simulink model "MVDR_example_hdl_4x4_systolic"  (R2020a)
settings: Solver=FixedStepDiscrete  StartTime=0.0  StopTime=stoptime  RelTol=1e-3
InitFcn:
  | model_init
values from neighbouring files (symbols this model uses):
  BackSubstitutePrototype = fi(0, matrixdivbacksub_dt)    [model_init.m]
  matrixDivDelay = NumberOfCORDICIterations*10 + 86    [model_init.m]
  movavg_bitshift = nextpow2(sqrt(windowSize))    [model_init.m]
  mvdrPipelineDelay = covMatDelay+movAvgDelay+matrixDivDelay+normResponseDelay    [model_init.m]
  numArrayElements = 4    [model_init.m]
  NumberOfCORDICIterations = matrixdivin_dt.WordLength - 1    [model_init.m]
  srcAngles = [20 60]    [model_init.m]
  sv = step(steeringVector,fc,[scanAngle; 0])    [model_init.m]
  Ts = 1/fs    (= 7.8125e-09)    [model_init.m]
  windowSize = 1024    [model_init.m]
libraries: hdlsllib x249, simulink x44, commfilt2 x4, commrfcorlib x3, commsync2 x3, commrflib2 x2, commrandsrc3 x2, phasedtxrxlib x2, commdigbbndcpm2 x1, dspsolvers x1, embreciprocals x1, commdigbbndpm3 x1
(part 1 of 11)
Description:
  | MVDR HDL 4x4 systolic testbench
settings Model: DataTypeOverride=Off  Creator=The MathWorks, Inc.  LastModifiedBy=tmealey
settings DataIOCC: LimitDataPoints=on  SaveFormat=Array  SaveOutput=off  SaveTime=off  ReturnWorkspaceOutputs=off
settings OptimizationCC: BlockReduction=off  ConditionallyExecuteInputs=off  DefaultParameterBehavior=Inlined  LifeSpan=inf
settings DebuggingCC: ReadBeforeWriteMsg=DisableAll  WriteAfterWriteMsg=DisableAll  WriteAfterReadMsg=DisableAll  AlgebraicLoopMsg=error  UnderspecifiedInitializationDetection=Classic  MergeDetectMultiDrivingBlocksExec=none  SolverPrmCheckMsg=warning  SingleTaskRateTransMsg=error  ParameterPrecisionLossMsg=none  AllowSymbolicDim=off  SFUnexpectedBacktrackingDiag=warning  SFNoUnconditionalDefaultTransitionDiag=warning  SFExecutionAtInitializationDiag=none  ArithmeticOperatorsInVariantConditions=warning
settings HardwareCC: ProdBitPerPointer=32  ProdBitPerSizeT=32  ProdBitPerPtrDiffT=32  ProdLargestAtomicFloat=None  ProdIntDivRoundTo=Undefined  ProdEndianess=Unspecified  ProdWordSize=32  ProdHWDeviceType=ASIC/FPGA->ASIC/FPGA  TargetBitPerPointer=64  TargetBitPerSizeT=64  TargetBitPerPtrDiffT=64  TargetLongLongMode=on  TargetIntDivRoundTo=Zero  TargetEndianess=LittleEndian  TargetWordSize=64  TargetHWDeviceType=Custom Processor->MATLAB Host Computer  ProdEqTarget=off
settings ModelReferenceCC: PropagateSignalLabelsOutOfModel=off
settings SFSimCC: SimUseLocalCustomCode=off  CustomCodeUndefinedFunction=UseInterfaceOnly
settings RTWCC: RTWUseLocalCustomCode=off
settings CodeAppCC: StateflowObjectComments=on
settings GRTTargetCC: TargetLangStandard=C89/C90 (ANSI)
settings ConfigComp: CovMetricSettings=dw  CovHtmlReporting=on  CovSaveCumulativeToWorkspaceVar=on  CovSaveSingleToWorkspaceVar=on  CovExternalEMLEnable=off  CovSFcnEnable=off

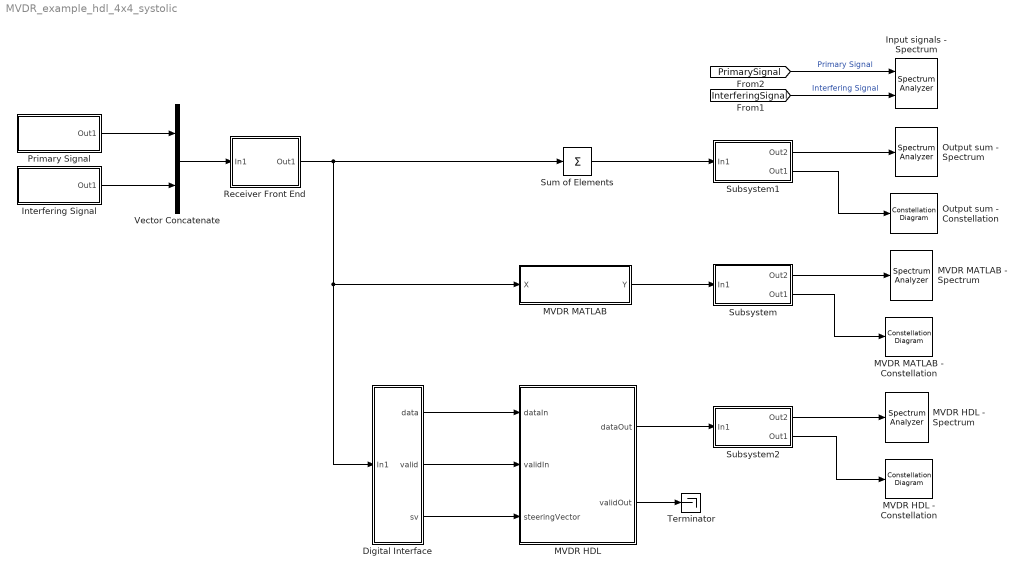
== system MVDR_example_hdl_4x4_systolic ==
  Digital Interface : Subsystem
  Input signals - Spectrum : SpectrumAnalyzer  NumInputPorts=2
  Interfering Signal : Subsystem
      mask Display: disp('Interfering\nSignal')
  MVDR HDL : Subsystem
  MVDR HDL - Constellation : ConstellationDiagram
  MVDR HDL - Spectrum : SpectrumAnalyzer
  MVDR MATLAB : Subsystem
  MVDR MATLAB - Constellation : ConstellationDiagram
  MVDR MATLAB - Spectrum : SpectrumAnalyzer
  Output sum - Constellation : ConstellationDiagram
  Output sum - Spectrum : SpectrumAnalyzer
  Primary Signal : Subsystem
      mask Display: disp('Primary\nSignal')
  Receiver Front End : Subsystem
  Subsystem : Subsystem
  Subsystem1 : Subsystem
  Subsystem2 : Subsystem
  Sum of Elements : Sum  Inputs=+  CollapseMode=Specified dimension  CollapseDim=2
  Terminator : Terminator
  Vector Concatenate : Concatenate  Mode=Multidimensional array  ConcatenateDimension=2
  wires:
  MVDR HDL/2(validOut) -> Terminator/1
  MVDR MATLAB/1(Y) -> Subsystem/1(In1)
  Interfering Signal/1(Out1) -> Vector Concatenate/2
  Primary Signal/1(Out1) -> Vector Concatenate/1
  [InterferingSignal] -> Input signals - Spectrum/2  "Interfering Signal"
  Subsystem/2(Out1) -> MVDR MATLAB - Constellation/1
  Subsystem/1(Out2) -> MVDR MATLAB - Spectrum/1
  Sum of Elements/1 -> Subsystem1/1(In1)
  Subsystem1/1(Out2) -> Output sum - Spectrum/1
  Subsystem1/2(Out1) -> Output sum - Constellation/1
  MVDR HDL/1(dataOut) -> Subsystem2/1(In1)
  Subsystem2/1(Out2) -> MVDR HDL - Spectrum/1
  Subsystem2/2(Out1) -> MVDR HDL - Constellation/1
  [PrimarySignal] -> Input signals - Spectrum/1  "Primary Signal"
  Digital Interface/1(data) -> MVDR HDL/1(dataIn)
  Digital Interface/2(valid) -> MVDR HDL/2(validIn)
  Digital Interface/3(sv) -> MVDR HDL/3(steeringVector)
  Receiver Front End/1(Out1) -> MVDR MATLAB/1(X), Digital Interface/1(In1), Sum of Elements/1
  Vector Concatenate/1 -> Receiver Front End/1(In1)

== system MVDR_example_hdl_4x4_systolic/Digital Interface ==
  In1 : Inport
  Constant1 : Constant  Value=true  SampleTime=-1
  Constant2 : Constant  Value=sv  SampleTime=-1
  Data Type Conversion : DataTypeConversion  OutDataTypeStr=sv_dt
  Input DTC : Subsystem
  Reshape : Reshape  OutputDimensionality=Column vector (2-D)
  Unbuffer : Unbuffer
  data : Outport
  valid : Outport  Port=2
  sv : Outport  Port=3
  wires:
  Unbuffer/1 -> Input DTC/1(In1)
  Constant2/1 -> Data Type Conversion/1
  In1/1 -> Unbuffer/1
  Data Type Conversion/1 -> Reshape/1
  Constant1/1 -> valid/1
  Input DTC/1(Out1) -> data/1
  Reshape/1 -> sv/1

== system MVDR_example_hdl_4x4_systolic/Interfering Signal ==
  GMSK Modulator Baseband : commdigbbndcpm2/GMSK Modulator Baseband  inputType=Bit  BT=.3  pulseLength=4  preHistory=1  phaseOffset=0  samplesPerSymbol=8  RateOptions=Enforce single-rate processing  outDataType=double
      settings: SourceProductBaseCode=CM
  Gain : Gain  Gain=1/40
  Memoryless Nonlinearity2 : commrflib2/Memoryless Nonlinearity  model_select=Cubic polynomial  linGaindB=39  GindB=0  iip3=43  am2pm=.8  LPwrLimAMPM=-2.5  UPwrLimAMPM=17.5  amam=[2.1587 1.1517]  ampm=[4.0033 9.1040]  x=[8.1081 1.5413 6.5202 -0.0718]  y=[4.6645 2.0965 10.88 -0.003]  p=0.5  GoutdB=0  vsat=1
      settings: SourceProductBaseCode=CM
  Random Integer Generator1 : commrandsrc3/Random Integer Generator  SetSize=2  SeedSource=Auto  Seed=0  SampleTime=4*Ts  SamplesPerFrame=100  OutputDataType=boolean  SimulateUsing=Interpreted execution
  Out1 : Outport  VectorParamsAs1DForOutWhenUnconnected=off
  tag scope: InterferingSignal=global
  wires:
  Memoryless Nonlinearity2/1 -> Gain/1
  GMSK Modulator Baseband/1 -> Memoryless Nonlinearity2/1
  Random Integer Generator1/1 -> GMSK Modulator Baseband/1
  Gain/1 -> Out1/1, [InterferingSignal]

== system MVDR_example_hdl_4x4_systolic/MVDR HDL ==
  dataIn : Inport
  validIn : Inport  Port=2
  steeringVector : Inport  Port=3
  Compute Weight Vector : Subsystem
  Form Beam : Subsystem
  Form Covariance Matrix : Subsystem
  Moving Average : Subsystem
  Normalize Response : Subsystem
  dataOut : Outport
  validOut : Outport  Port=2
  wires:
  Normalize Response/1(wOut) -> Form Beam/3(w)
  Form Beam/1(dataOut) -> dataOut/1
  Form Covariance Matrix/2(validOut) -> Moving Average/2(validIn)
  Form Beam/2(validOut) -> validOut/1
  Compute Weight Vector/1(w) -> Normalize Response/1(wIn)
  steeringVector/1 -> Compute Weight Vector/3(steeringVector), Normalize Response/3(steeringVector)
  Form Covariance Matrix/1(dataOut) -> Moving Average/1(dataIn)
  Moving Average/1(dataOut) -> Compute Weight Vector/1(covarianceMatrix)
  Moving Average/2(validOut) -> Compute Weight Vector/2(validIn)
  Compute Weight Vector/2(validOut) -> Normalize Response/2(validIn)
  dataIn/1 -> Form Covariance Matrix/1(dataIn), Form Beam/1(dataIn)
  validIn/1 -> Form Covariance Matrix/2(validIn), Form Beam/2(validIn)

== system MVDR_example_hdl_4x4_systolic/MVDR MATLAB ==
  X : Inport
  MATLAB Function : MATLAB Function  TreatAsAtomicUnit=on
  Y : Outport
  wires:
  MATLAB Function/1(Y) -> Y/1
  X/1 -> MATLAB Function/1(X)

== system MVDR_example_hdl_4x4_systolic/Primary Signal ==
  Gain : Gain  Gain=1/40
  Memoryless Nonlinearity : commrflib2/Memoryless Nonlinearity  model_select=Cubic polynomial  linGaindB=28  GindB=0  iip3=43  am2pm=.8  LPwrLimAMPM=-2.5  UPwrLimAMPM=17.5  amam=[2.1587 1.1517]  ampm=[4.0033 9.1040]  x=[8.1081 1.5413 6.5202 -0.0718]  y=[4.6645 2.0965 10.88 -0.003]  p=0.5  GoutdB=0  vsat=1
      settings: SourceProductBaseCode=CM
  QPSK Modulator Baseband : commdigbbndpm3/QPSK Modulator Baseband  InType=Integer  Enc=Gray  Ph=pi/4  outDtype=double  outWordLen=16  outUDDataType=sfix(16)  outFracLenMode=Best precision  outFracLen=15  outDataTypeStr=double  outLastDataTypeStr=double
  Raised Cosine Transmit Filter : commfilt2/Raised Cosine Transmit Filter  filtType=Square root  R=.3  filtSpan=10  N=2  filterGain=1  InputProcessing=Columns as channels (frame based)  RateOptions=Enforce single-rate processing  framing=Mute  checkCoeff=off  variableName=rcTxFilt  checkGain=Normalized  sampMode=Mute  saveAsFlag=0  currentFiltSpan=10  D=(10)/2  launchFVT=on  roundingMode=Floor  overflowMode=off  coeffDataTypeStr=Inherit: Same word length as input  coeffMin=[]  coeffMax=[]  coeffLastDataTypeStr=Inherit: Same word length as input  outputDataTypeStr=Inherit: Same as accumulator  outputMin=[]  outputMax=[]  outputLastDataTypeStr=Inherit: Same as accumulator
  Random Integer Generator : commrandsrc3/Random Integer Generator  SetSize=4  SeedSource=Auto  Seed=0  SampleTime=Ts  SamplesPerFrame=400  OutputDataType=double  SimulateUsing=Interpreted execution
  Out1 : Outport  VectorParamsAs1DForOutWhenUnconnected=off
  tag scope: PrimarySignal=global
  wires:
  QPSK Modulator Baseband/1 -> Raised Cosine Transmit Filter/1
  Random Integer Generator/1 -> QPSK Modulator Baseband/1
  Memoryless Nonlinearity/1 -> Gain/1
  Raised Cosine Transmit Filter/1 -> Memoryless Nonlinearity/1
  Gain/1 -> Out1/1, [PrimarySignal]

== system MVDR_example_hdl_4x4_systolic/Receiver Front End ==
  In1 : Inport
  Constant : Constant  Value=srcAngles  SampleTime=-1
  Narrowband Receive Array : phasedtxrxlib/Narrowband Receive Array  PropagationSpeed=propSpeed  OperatingFrequency=fc  Wavefront=Plane  SensorGainMeasure=dB  Polarization=None  WeightsInputPort=off  SimulateUsing=Interpreted execution  Sensor=sensorArray
      settings: SourceProductBaseCode=AR
  Receiver Preamp : phasedtxrxlib/Receiver Preamp  Gain=-10  LossFactor=0  NoiseMethod=Noise power  NoiseFigure=0  ReferenceTemperature=290  SampleRateFromInputCheckbox=on  SampleRate=1e6  NoisePower=.001  EnableInputPort=off  PhaseNoiseInputPort=off  SeedSource=Auto  Seed=0  SimulateUsing=Interpreted execution
      settings: SourceProductBaseCode=AR
  Reshape : Reshape  OutputDimensionality=Row vector (2-D)
  Out1 : Outport
  wires:
  In1/1 -> Narrowband Receive Array/1
  Narrowband Receive Array/1 -> Receiver Preamp/1
  Constant/1 -> Reshape/1
  Reshape/1 -> Narrowband Receive Array/2
  Receiver Preamp/1 -> Out1/1

== system MVDR_example_hdl_4x4_systolic/Subsystem ==
  In1 : Inport
  AGC : commrfcorlib/AGC  LegacyMode=off  DetectorMethod=Rectifier  LoopMethod=Linear  UpdatePeriod=100  StepSize=0.1  AdaptationStepSize=0.01  DesiredOutputPower=1  AveragingLength=200  MaximumGain=30  MaxPowerGain=60  GainOutputPort=off  InputPowerOutputPort=off  SimulateUsing=Interpreted execution
  Carrier Synchronizer : commsync2/Carrier Synchronizer  Modulation=QPSK  ModulationPhaseOffset=Auto  CustomPhaseOffset=0  SamplesPerSymbol=1  DampingFactor=0.707  NormalizedLoopBandwidth=0.01  EstimatedPhaseErrorOutputPort=off  SimulateUsing=Interpreted execution
  Raised Cosine Receive Filter : commfilt2/Raised Cosine Receive Filter  filtType=Square root  R=.3  filtSpan=10  N=2  downFactor=2  downOffset=0  filterGain=1  InputProcessing=Columns as channels (frame based)  RateOptions=Enforce single-rate processing  framing=Mute  checkCoeff=off  variableName=rcRxFilt  currentFiltSpan=10  D=5  inputOffset=0  sampMode=Mute  saveAsFlag=0  rateMode=Downsampling  checkGain=Normalized  launchFVT=on  roundingMode=Floor  overflowMode=off  coeffDataTypeStr=Inherit: Same word length as input  coeffMin=[]  coeffMax=[]  coeffLastDataTypeStr=Inherit: Same word length as input  accumDataTypeStr=Inherit: Same as product output  accumLastDataTypeStr=Inherit: Same as product output  outputDataTypeStr=Inherit: Same as accumulator  outputMin=[]  outputMax=[]  outputLastDataTypeStr=Inherit: Same as accumulator
  Out2 : Outport
  Out1 : Outport  Port=2
  wires:
  In1/1 -> Out2/1, Raised Cosine Receive Filter/1
  Raised Cosine Receive Filter/1 -> Carrier Synchronizer/1
  AGC/1 -> Out1/1
  Carrier Synchronizer/1 -> AGC/1

== system MVDR_example_hdl_4x4_systolic/Subsystem1 ==
  In1 : Inport
  AGC : commrfcorlib/AGC  LegacyMode=off  DetectorMethod=Rectifier  LoopMethod=Linear  UpdatePeriod=100  StepSize=0.1  AdaptationStepSize=0.01  DesiredOutputPower=1  AveragingLength=200  MaximumGain=30  MaxPowerGain=60  GainOutputPort=off  InputPowerOutputPort=off  SimulateUsing=Interpreted execution
  Carrier Synchronizer : commsync2/Carrier Synchronizer  Modulation=QPSK  ModulationPhaseOffset=Auto  CustomPhaseOffset=0  SamplesPerSymbol=1  DampingFactor=0.707  NormalizedLoopBandwidth=0.01  EstimatedPhaseErrorOutputPort=off  SimulateUsing=Interpreted execution
  Raised Cosine Receive Filter : commfilt2/Raised Cosine Receive Filter  filtType=Square root  R=.3  filtSpan=10  N=2  downFactor=2  downOffset=0  filterGain=1  InputProcessing=Columns as channels (frame based)  RateOptions=Enforce single-rate processing  framing=Mute  checkCoeff=off  variableName=rcRxFilt  currentFiltSpan=10  D=5  inputOffset=0  sampMode=Mute  saveAsFlag=0  rateMode=Downsampling  checkGain=Normalized  launchFVT=on  roundingMode=Floor  overflowMode=off  coeffDataTypeStr=Inherit: Same word length as input  coeffMin=[]  coeffMax=[]  coeffLastDataTypeStr=Inherit: Same word length as input  accumDataTypeStr=Inherit: Same as product output  accumLastDataTypeStr=Inherit: Same as product output  outputDataTypeStr=Inherit: Same as accumulator  outputMin=[]  outputMax=[]  outputLastDataTypeStr=Inherit: Same as accumulator
  Out2 : Outport
  Out1 : Outport  Port=2
  wires:
  Carrier Synchronizer/1 -> AGC/1
  AGC/1 -> Out1/1
  Raised Cosine Receive Filter/1 -> Carrier Synchronizer/1
  In1/1 -> Raised Cosine Receive Filter/1, Out2/1

== system MVDR_example_hdl_4x4_systolic/Subsystem2 ==
  In1 : Inport
  AGC : commrfcorlib/AGC  LegacyMode=off  DetectorMethod=Rectifier  LoopMethod=Linear  UpdatePeriod=100  StepSize=0.1  AdaptationStepSize=0.01  DesiredOutputPower=1  AveragingLength=200  MaximumGain=30  MaxPowerGain=60  GainOutputPort=off  InputPowerOutputPort=off  SimulateUsing=Interpreted execution
  Buffer : Buffer  N=800  OutputFrames=off
  Carrier Synchronizer : commsync2/Carrier Synchronizer  Modulation=QPSK  ModulationPhaseOffset=Auto  CustomPhaseOffset=0  SamplesPerSymbol=1  DampingFactor=0.707  NormalizedLoopBandwidth=0.01  EstimatedPhaseErrorOutputPort=off  SimulateUsing=Interpreted execution
  Data Type Conversion : DataTypeConversion  OutDataTypeStr=double
  Raised Cosine Receive Filter : commfilt2/Raised Cosine Receive Filter  filtType=Square root  R=.3  filtSpan=10  N=2  downFactor=2  downOffset=0  filterGain=1  InputProcessing=Columns as channels (frame based)  RateOptions=Enforce single-rate processing  framing=Mute  checkCoeff=off  variableName=rcRxFilt  currentFiltSpan=10  D=5  inputOffset=0  sampMode=Mute  saveAsFlag=0  rateMode=Downsampling  checkGain=Normalized  launchFVT=on  roundingMode=Floor  overflowMode=off  coeffDataTypeStr=Inherit: Same word length as input  coeffMin=[]  coeffMax=[]  coeffLastDataTypeStr=Inherit: Same word length as input  accumDataTypeStr=Inherit: Same as product output  accumLastDataTypeStr=Inherit: Same as product output  outputDataTypeStr=Inherit: Same as accumulator  outputMin=[]  outputMax=[]  outputLastDataTypeStr=Inherit: Same as accumulator
  Out2 : Outport
  Out1 : Outport  Port=2
  wires:
  Carrier Synchronizer/1 -> AGC/1
  AGC/1 -> Out1/1
  Raised Cosine Receive Filter/1 -> Carrier Synchronizer/1
  In1/1 -> Buffer/1
  Data Type Conversion/1 -> Raised Cosine Receive Filter/1, Out2/1
  Buffer/1 -> Data Type Conversion/1

== system MVDR_example_hdl_4x4_systolic/Digital Interface/Input DTC ==
  In1 : Inport
  Data Type Conversion : DataTypeConversion  OutDataTypeStr=input_dt
  Data Type Conversion1 : DataTypeConversion  OutDataTypeStr=adc_dt
  Out1 : Outport
  wires:
  Data Type Conversion/1 -> Out1/1
  In1/1 -> Data Type Conversion1/1
  Data Type Conversion1/1 -> Data Type Conversion/1

== system MVDR_example_hdl_4x4_systolic/MVDR HDL/Compute Weight Vector ==
  covarianceMatrix : Inport
  validIn : Inport  Port=2
  steeringVector : Inport  Port=3
  Data Type Conversion1 : DataTypeConversion  OutDataTypeStr=matrixdivin_dt
  Data Type Conversion2 : DataTypeConversion  OutDataTypeStr=matrixdivin_dt
  Data Type Conversion3 : DataTypeConversion  OutDataTypeStr=matrixdivout_dt
  Delay : Delay  DelayLength=1
  Logical Operator : Logic  IconShape=distinctive  AllPortsSameDT=off  OutDataTypeStr=boolean
  Matrix Left Divide : Subsystem  Variant=on  VariantControlMode=Label  LabelModeActiveChoice=HDL
  w : Outport
  validOut : Outport  Port=2
  wires:
  covarianceMatrix/1 -> Data Type Conversion1/1
  steeringVector/1 -> Data Type Conversion2/1
  Data Type Conversion3/1 -> w/1
  Data Type Conversion1/1 -> Matrix Left Divide/1(A)
  Data Type Conversion2/1 -> Matrix Left Divide/2(B)
  Matrix Left Divide/3(ready) -> Delay/1
  Matrix Left Divide/1(x) -> Data Type Conversion3/1
  validIn/1 -> Logical Operator/1
  Logical Operator/1 -> Matrix Left Divide/3(validIn)
  Delay/1 -> Logical Operator/2
  Matrix Left Divide/2(validOut) -> validOut/1

== system MVDR_example_hdl_4x4_systolic/MVDR HDL/Form Beam ==
  dataIn : Inport
  validIn : Inport  Port=2
  w : Inport  Port=3
  Data Type Conversion : DataTypeConversion  OutDataTypeStr=output_dt
  Delay1 : Delay  DelayLength=6
  Delay2 : Delay
  Delay3 : Delay  DelayLength=mvdrPipelineDelay
  Delay7 : Delay  DelayLength=mvdrPipelineDelay
  Math Function2 : Math  Operator=conj  SaturateOnIntegerOverflow=on
  Parallel Complex Multiply : Subsystem  TreatAsAtomicUnit=on
  Reshape : Reshape
  Reshape1 : Reshape
  Tree Sum : Subsystem
  dataOut : Outport
  validOut : Outport  Port=2
  wires:
  dataIn/1 -> Delay7/1
  Parallel Complex Multiply/1(z) -> Tree Sum/1(In1)
  Tree Sum/1(Out1) -> Data Type Conversion/1
  Math Function2/1 -> Reshape/1
  w/1 -> Math Function2/1
  validIn/1 -> Delay3/1
  Reshape/1 -> Parallel Complex Multiply/2(z2)
  Reshape1/1 -> Parallel Complex Multiply/1(z1)
  Data Type Conversion/1 -> dataOut/1
  Delay2/1 -> validOut/1
  Delay1/1 -> Delay2/1
  Delay3/1 -> Delay1/1
  Delay7/1 -> Reshape1/1

== system MVDR_example_hdl_4x4_systolic/MVDR HDL/Form Covariance Matrix ==
  dataIn : Inport
  validIn : Inport  Port=2
  Conj : Math  Operator=conj
  Data Type Conversion : DataTypeConversion  OutDataTypeStr=covmat_dt
  Data Type Conversion1 : DataTypeConversion  OutDataTypeStr=adc_dt
  Delay : Delay  DelayLength=6
  Matrix Multiply Partitioned : Subsystem  TreatAsAtomicUnit=on
  Reshape : Reshape
  dataOut : Outport
  validOut : Outport  Port=2
  wires:
  validIn/1 -> Delay/1
  dataIn/1 -> Data Type Conversion1/1
  Reshape/1 -> Conj/1, Matrix Multiply Partitioned/1(x)  "x"
  Matrix Multiply Partitioned/1(C) -> Data Type Conversion/1  "x * x'"
  Delay/1 -> validOut/1
  Conj/1 -> Matrix Multiply Partitioned/2(x_conj)
  Data Type Conversion1/1 -> Reshape/1
  Data Type Conversion/1 -> dataOut/1

== system MVDR_example_hdl_4x4_systolic/MVDR HDL/Moving Average ==
  note: Shift replaces gain by 1/sqrt(windowSize)
  dataIn : Inport
  validIn : Inport  Port=2
  Add : Sum  Inputs=++-  AccumDataTypeStr=movavg_accum_dt  OutDataTypeStr=Inherit: Same as accumulator
  Bit Shift : hdlsllib/Logic and Bit Operations/Bit Shift  mode=Shift Right Arithmetic  N=movavg_bitshift
  Data Type Conversion : DataTypeConversion  OutDataTypeStr=movavg_out_dt
  Delay : Delay  DelayLength=windowSize
  Delay{1..5} (5 alike) : Delay  DelayLength=1
  Reshape : Reshape
  Reshape1 : Reshape  OutputDimensionality=Customize  OutputDimensions=[4,4]
  Wait for Running Sum Init : Subsystem
  dataOut : Outport
  validOut : Outport  Port=2
  wires:
  Bit Shift/1 -> Data Type Conversion/1
  Delay1/1 -> Bit Shift/1, Add/1
  Delay/1 -> Add/3
  Add/1 -> Delay1/1
  dataIn/1 -> Reshape/1
  validIn/1 -> Delay3/1
  Delay2/1 -> Delay/1, Add/2
  Delay4/1 -> Reshape1/1
  Delay5/1 -> validOut/1
  Data Type Conversion/1 -> Delay4/1
  Delay3/1 -> Wait for Running Sum Init/1(In1)
  Wait for Running Sum Init/1(Out1) -> Delay5/1
  Reshape/1 -> Delay2/1
  Reshape1/1 -> dataOut/1

== system MVDR_example_hdl_4x4_systolic/MVDR HDL/Normalize Response ==
  note: This subsystem scales the weight vector to ensure unit gain in the target direction.
  wIn : Inport
  validIn : Inport  Port=2
  steeringVector : Inport  Port=3
  MVDR Weight Update : Subsystem
  Unit Delay Enabled Synchronous : hdlsllib/Discrete/Unit Delay Enabled Synchronous  InitialCondition=0.0  SampleTime=-1
      settings: SourceProductBaseCode=SL
  wOut : Outport
  wires:
  steeringVector/1 -> MVDR Weight Update/1(Steering Vector)
  wIn/1 -> MVDR Weight Update/2(x)
  MVDR Weight Update/1(w) -> Unit Delay Enabled Synchronous/1
  MVDR Weight Update/2(validOut) -> Unit Delay Enabled Synchronous/2
  Unit Delay Enabled Synchronous/1 -> wOut/1
  validIn/1 -> MVDR Weight Update/3(validIn)

== system MVDR_example_hdl_4x4_systolic/MVDR HDL/Compute Weight Vector/Matrix Left Divide ==
  A : Inport
  B : Inport  Port=2
  validIn : Inport  Port=3
  CORDIC : Subsystem  VariantControl=HDL
  QR Solver : Subsystem  VariantControl=Simulation
  x : Outport
  validOut : Outport  Port=2
  ready : Outport  Port=3

== system MVDR_example_hdl_4x4_systolic/MVDR HDL/Form Beam/Parallel Complex Multiply ==
  z1 : Inport  Partition=on  PartitionDimension=1  PartitionWidth=1  PartitionOffset=0
  z2 : Inport  Port=2  Partition=on  PartitionDimension=1  PartitionWidth=1  PartitionOffset=0
  For Each : ForEach  DisableCoverage=on
  HDL Complex Multiply : Subsystem  mask(HDL Complex Multiplier (3 Multiply, 5 Add)){D1=2, D2=1, D3=1, D4=1, D5=1}
      mask help:
      | Xilinx devices:
      | - Set D1 = 1 or 2 to trade off speed & FF resources
      | - Set D2-D5 = 1 to fully leverage DSP48 pipelines
      | - Use sync reset
      |
      | Intel FPGAs:
      | - Set D1 = 1 or 2 depending on device family
      | - Set D5 = 1; D2, D3, D4 = 0
      | - Use async reset
      mask init:
      | delay = D1+D2+D3+D4+D5;
      mask Display:
      | fprintf('Delay=%d',delay);
      | port_label('input',1,'z1');
      | port_label('input',2,'z2');
  z : Outport  ConcatenationDimension=1
  wires:
  z1/1 -> HDL Complex Multiply/1(In1)
  z2/1 -> HDL Complex Multiply/2(In2)
  HDL Complex Multiply/1(Out1) -> z/1

== system MVDR_example_hdl_4x4_systolic/MVDR HDL/Form Beam/Tree Sum ==
  In1 : Inport
  Delay3 : Delay  DelayLength=ceil(log2(numArrayElements))
  Tree Sum of Elements : Sum  Inputs=+  OutDataTypeStr=Inherit: Same as first input  LockScale=on
  Out1 : Outport
  wires:
  Delay3/1 -> Out1/1
  In1/1 -> Tree Sum of Elements/1
  Tree Sum of Elements/1 -> Delay3/1

== system MVDR_example_hdl_4x4_systolic/MVDR HDL/Form Covariance Matrix/Matrix Multiply Partitioned ==
  x : Inport
  x_conj : Inport  Port=2
  Partition x_conj : Subsystem
  Reshape : Reshape  OutputDimensionality=Customize  OutputDimensions=[4,4]
  C : Outport
  wires:
  x/1 -> Partition x_conj/1(x)
  x_conj/1 -> Partition x_conj/2(x_conj)
  Partition x_conj/1(C) -> Reshape/1
  Reshape/1 -> C/1

== system MVDR_example_hdl_4x4_systolic/MVDR HDL/Moving Average/Wait for Running Sum Init ==
  In1 : Inport
  Compare To Constant : simulink/Logic and Bit Operations/Compare To Constant  relop=<  const=windowSize  OutDataTypeStr=boolean
  HDL Counter : hdlsllib/Sources/HDL Counter  CountType=Free running  CountInit=0  CountStep=1  CountMax=25  CountFromType=Initial value  CountFrom=0  CountResetPort=off  CountLoadPort=off  CountEnbPort=on  CountDirPort=off  CountDataType=Unsigned  CountWordLen=nextpow2(windowSize)+1  CountFracLen=0  CountSampTime=1
  Logical Operator : Logic  IconShape=distinctive  AllPortsSameDT=off  OutDataTypeStr=boolean
  Logical Operator1 : Logic  IconShape=distinctive  AllPortsSameDT=off  OutDataTypeStr=boolean
  Logical Operator2 : Logic  Operator=NOT  IconShape=distinctive  AllPortsSameDT=off  OutDataTypeStr=boolean
  Out1 : Outport
  wires:
  Logical Operator2/1 -> Logical Operator/2
  Logical Operator1/1 -> HDL Counter/1
  Compare To Constant/1 -> Logical Operator1/2, Logical Operator2/1
  Logical Operator/1 -> Out1/1
  HDL Counter/1 -> Compare To Constant/1
  In1/1 -> Logical Operator1/1, Logical Operator/1

== system MVDR_example_hdl_4x4_systolic/MVDR HDL/Normalize Response/MVDR Weight Update ==
  Steering Vector : Inport
  x : Inport  Port=2
  validIn : Inport  Port=3
  Delay{,1,3..6} (6 alike) : Delay  DelayLength=1
  Delay2 : Delay  DelayLength=8
  Inner Product : Subsystem
  Vector / Scalar Divide : Subsystem
  w : Outport
  validOut : Outport  Port=2
  wires:
  x/1 -> Delay3/1
  Vector / Scalar Divide/1(w) -> w/1
  Delay4/1 -> Inner Product/1(u)
  Inner Product/1(y) -> Delay5/1
  Delay6/1 -> Vector / Scalar Divide/1(x)
  Delay/1 -> Vector / Scalar Divide/3(validIn)
  Steering Vector/1 -> Delay4/1
  Delay3/1 -> Delay2/1, Inner Product/2(v)
  Delay5/1 -> Vector / Scalar Divide/2(y)
  Inner Product/2(validOut) -> Delay/1
  validIn/1 -> Delay1/1
  Vector / Scalar Divide/2(validOut) -> validOut/1
  Delay1/1 -> Inner Product/3(validIn)
  Delay2/1 -> Delay6/1

== system MVDR_example_hdl_4x4_systolic/MVDR HDL/Compute Weight Vector/Matrix Left Divide/CORDIC ==
  A : Inport
  B : Inport  Port=2
  validIn : Inport  Port=3
  4x4 Complex CORDIC Matrix Left Divide : Subsystem  TreatAsAtomicUnit=on  mask(4x4 Complex CORDIC Matrix Left Divide){NumberOfCORDICIterations=NumberOfCORDICIterations, OutputPrototype=BackSubstitutePrototype}
      mask prompts: NumberOfCORDICIterations "Number of CORDIC Iterations"; OutputPrototype "Back-Substitute Prototype"
      mask help: Solve AX=B using QR factorization using CORDIC. Matrix A must be 4x4. Matrix B must have 4 rows.
  Demux : Demux
  Selector : Selector  NumberOfDimensions=2  InputPortWidth=3  IndexOptions=Index vector (dialog),Select all  Indices=1,1  OutputSizes=1,1
  Selector1 : Selector  NumberOfDimensions=2  InputPortWidth=3  IndexOptions=Index vector (dialog),Select all  Indices=2,1  OutputSizes=1,1
  Selector2 : Selector  NumberOfDimensions=2  InputPortWidth=3  IndexOptions=Index vector (dialog),Select all  Indices=3,1  OutputSizes=1,1
  Selector3 : Selector  NumberOfDimensions=2  InputPortWidth=3  IndexOptions=Index vector (dialog),Select all  Indices=4,1  OutputSizes=1,1
  Vector Concatenate : Concatenate  NumInputs=4  Mode=Multidimensional array
  x : Outport
  validOut : Outport  Port=2
  ready : Outport  Port=3
  wires:
  Selector/1 -> 4x4 Complex CORDIC Matrix Left Divide/1(a1)
  4x4 Complex CORDIC Matrix Left Divide/2(x2) -> Vector Concatenate/2
  4x4 Complex CORDIC Matrix Left Divide/1(x1) -> Vector Concatenate/1
  4x4 Complex CORDIC Matrix Left Divide/3(x3) -> Vector Concatenate/3
  4x4 Complex CORDIC Matrix Left Divide/4(x4) -> Vector Concatenate/4
  4x4 Complex CORDIC Matrix Left Divide/6(ready) -> ready/1
  Selector1/1 -> 4x4 Complex CORDIC Matrix Left Divide/2(a2)
  Selector2/1 -> 4x4 Complex CORDIC Matrix Left Divide/3(a3)
  Selector3/1 -> 4x4 Complex CORDIC Matrix Left Divide/4(a4)
  Demux/1 -> 4x4 Complex CORDIC Matrix Left Divide/5(b1)
  Demux/4 -> 4x4 Complex CORDIC Matrix Left Divide/8(b4)
  Demux/2 -> 4x4 Complex CORDIC Matrix Left Divide/6(b2)
  Demux/3 -> 4x4 Complex CORDIC Matrix Left Divide/7(b3)
  4x4 Complex CORDIC Matrix Left Divide/5(validOut) -> validOut/1
  A/1 -> Selector1/1, Selector2/1, Selector3/1, Selector/1
  B/1 -> Demux/1
  validIn/1 -> 4x4 Complex CORDIC Matrix Left Divide/9(validIn)
  Vector Concatenate/1 -> x/1

== system MVDR_example_hdl_4x4_systolic/MVDR HDL/Compute Weight Vector/Matrix Left Divide/QR Solver ==
  A : Inport
  B : Inport  Port=2
  validIn : Inport  Port=3
  Data Type Conversion : DataTypeConversion  OutDataTypeStr=single
  Data Type Conversion1 : DataTypeConversion  OutDataTypeStr=single
  Data Type Conversion2 : DataTypeConversion  OutDataTypeStr=matrixdivbacksub_dt
  Delay1 : Delay  DelayLength=matrixDivDelay
  Delay6 : Delay  DelayLength=matrixDivDelay
  Emulate CORDIC Ready : Subsystem
  Reshape : Reshape  OutputDimensionality=Customize  OutputDimensions=[4,4]
  Reshape1 : Reshape  OutputDimensionality=Customize  OutputDimensions=[4,1]
  Subsystem : Subsystem
  x : Outport
  validOut : Outport  Port=2
  ready : Outport  Port=3
  wires:
  B/1 -> Reshape1/1
  A/1 -> Reshape/1
  validIn/1 -> Emulate CORDIC Ready/1(In1), Subsystem/Enable, Delay1/1
  Reshape/1 -> Data Type Conversion/1
  Emulate CORDIC Ready/1(Out1) -> ready/1
  Delay6/1 -> Data Type Conversion2/1
  Delay1/1 -> validOut/1
  Data Type Conversion/1 -> Subsystem/1(In1)
  Data Type Conversion1/1 -> Subsystem/2(In2)
  Subsystem/1(Out1) -> Delay6/1
  Reshape1/1 -> Data Type Conversion1/1
  Data Type Conversion2/1 -> x/1

== system MVDR_example_hdl_4x4_systolic/MVDR HDL/Form Beam/Parallel Complex Multiply/HDL Complex Multiply ==
  note: Xilinx devices:
      | - Set D1 = 1 or 2 to trade off speed & FF resources
      | - Set D2-D5 = 1 to fully leverage DSP48 pipelines
      | - Use sync reset
      |
      | Intel FPGAs:
      | - Set D1 = 1 or 2 depending on device family
      | - Set D5 = 1; D2, D3, D4 = 0
      | - Use async reset
  In1 : Inport
  In2 : Inport  Port=2
  Add1 : Sum
  Add2 : Sum  Inputs=+-
  Add3 : Sum
  Add4 : Sum  Inputs=-+
  Add5 : Sum
  Complex to Real-Imag : ComplexToRealImag
  Complex to Real-Imag1 : ComplexToRealImag
  D1_1 : Delay  DelayLength=D1
  D1_2 : Delay  DelayLength=D1
  D2_{1..6} (6 alike) : Delay  DelayLength=D2
  D3_{1..5} (5 alike) : Delay  DelayLength=D3
  D4_1 : Delay  DelayLength=D4
  D4_2 : Delay  DelayLength=D4
  D4_3 : Delay  DelayLength=D4
  D5_1 : Delay  DelayLength=D5
  D5_2 : Delay  DelayLength=D5
  Product1 : Product
  Product2 : Product
  Product3 : Product
  Real-Imag to Complex : RealImagToComplex
  Out1 : Outport  VectorParamsAs1DForOutWhenUnconnected=off
  wires:
  Real-Imag to Complex/1 -> Out1/1
  In2/1 -> D1_2/1
  Complex to Real-Imag1/1 -> Add3/1, D2_4/1  "C"
  Complex to Real-Imag1/2 -> Add3/2, D2_3/1  "D"
  Product1/1 -> D4_1/1  "X"
  Product2/1 -> D4_2/1  "Y"
  Product3/1 -> D3_5/1  "Z"
  Add4/1 -> D5_1/1
  Add5/1 -> D5_2/1
  D5_1/1 -> Real-Imag to Complex/1
  D5_2/1 -> Real-Imag to Complex/2
  D4_1/1 -> Add4/1
  D4_2/1 -> Add5/1
  D3_5/1 -> D4_3/1
  Add1/1 -> D3_1/1
  Add3/1 -> D2_6/1
  Add2/1 -> D3_3/1
  Complex to Real-Imag/1 -> D2_5/1, D2_1/1  "A"
  Complex to Real-Imag/2 -> D2_2/1  "B"
  D3_1/1 -> Product1/1
  D2_6/1 -> Product3/2
  D3_3/1 -> Product2/1
  D4_3/1 -> Add4/2, Add5/2
  D3_4/1 -> Product2/2
  D3_2/1 -> Product1/2
  D2_4/1 -> D3_4/1
  D2_3/1 -> D3_2/1
  D2_5/1 -> Product3/1
  D2_2/1 -> Add1/2, Add2/1
  D2_1/1 -> Add2/2, Add1/1
  In1/1 -> D1_1/1
  D1_1/1 -> Complex to Real-Imag/1
  D1_2/1 -> Complex to Real-Imag1/1

== system MVDR_example_hdl_4x4_systolic/MVDR HDL/Form Covariance Matrix/Matrix Multiply Partitioned/Partition x_conj ==
  x : Inport
  x_conj : Inport  Port=2  Partition=on  PartitionDimension=1  PartitionWidth=1  PartitionOffset=0
  For Each : ForEach  DisableCoverage=on
  Partition x : Subsystem  TreatAsAtomicUnit=on
  C : Outport  ConcatenationDimension=1
  wires:
  x_conj/1 -> Partition x/2(x_conj_elem)
  x/1 -> Partition x/1(x)
  Partition x/1(C_col) -> C/1

== system MVDR_example_hdl_4x4_systolic/MVDR HDL/Normalize Response/MVDR Weight Update/Inner Product ==
  u : Inport
  v : Inport  Port=2
  validIn : Inport  Port=3
  Conjugate : Math  Operator=conj  SignedPower=on  RndMeth=Zero  SaturateOnIntegerOverflow=on
  Delay : Delay  DelayLength=1
  Delay1 : Delay  DelayLength=6
  Delay2 : Delay  DelayLength=ceil(log2(numArrayElements))
  Delay4 : Delay  DelayLength=1
  Element-wise complex product : Subsystem  TreatAsAtomicUnit=on
  Tree Sum with Distributed Pipelining : Subsystem
  y : Outport
  validOut : Outport  Port=2
  wires:
  v/1 -> Conjugate/1
  u/1 -> Element-wise complex product/2(v)
  validIn/1 -> Delay1/1
  Element-wise complex product/1(y) -> Delay/1
  Delay2/1 -> validOut/1
  Delay1/1 -> Delay4/1
  Delay4/1 -> Delay2/1
  Conjugate/1 -> Element-wise complex product/1(u)
  Delay/1 -> Tree Sum with Distributed Pipelining/1(In1)
  Tree Sum with Distributed Pipelining/1(Out1) -> y/1

== system MVDR_example_hdl_4x4_systolic/MVDR HDL/Normalize Response/MVDR Weight Update/Vector // Scalar Divide ==
  x : Inport
  y : Inport  Port=2
  validIn : Inport  Port=3
  Complex to Real-Imag : ComplexToRealImag  Output=Real
  Data Type Conversion : DataTypeConversion  OutDataTypeStr=fixdt(1,18,16)
  Delay{1..6,11..13} (9 alike) : Delay  DelayLength=1
  Delay{7..10} (4 alike) : Delay
  Delay14 : Delay  DelayLength=34
  MATLAB Function : MATLAB Function  TreatAsAtomicUnit=on
  Normalized Reciprocal HDL Optimized : embreciprocals/Normalized Reciprocal HDL Optimized
      settings: SourceProductBaseCode=PO
  Product : Product  OutDataTypeStr=Inherit: Same as first input
  w : Outport
  validOut : Outport  Port=2
  wires:
  Delay2/1 -> MATLAB Function/2(e)
  y/1 -> Complex to Real-Imag/1
  Delay12/1 -> Data Type Conversion/1
  Complex to Real-Imag/1 -> Normalized Reciprocal HDL Optimized/1
  Delay13/1 -> Delay7/1
  Normalized Reciprocal HDL Optimized/2 -> Delay11/1
  Normalized Reciprocal HDL Optimized/1 -> Delay12/1
  Delay1/1 -> MATLAB Function/1(y)
  validIn/1 -> Normalized Reciprocal HDL Optimized/2
  Product/1 -> Delay1/1
  Delay11/1 -> Delay9/1
  MATLAB Function/1(w) -> Delay3/1
  Normalized Reciprocal HDL Optimized/3 -> Delay4/1
  Delay3/1 -> w/1
  Delay4/1 -> Delay10/1
  Delay5/1 -> Delay6/1
  Delay6/1 -> validOut/1
  x/1 -> Delay14/1
  Data Type Conversion/1 -> Delay8/1
  Delay7/1 -> Product/1
  Delay8/1 -> Product/2
  Delay9/1 -> Delay2/1
  Delay10/1 -> Delay5/1
  Delay14/1 -> Delay13/1

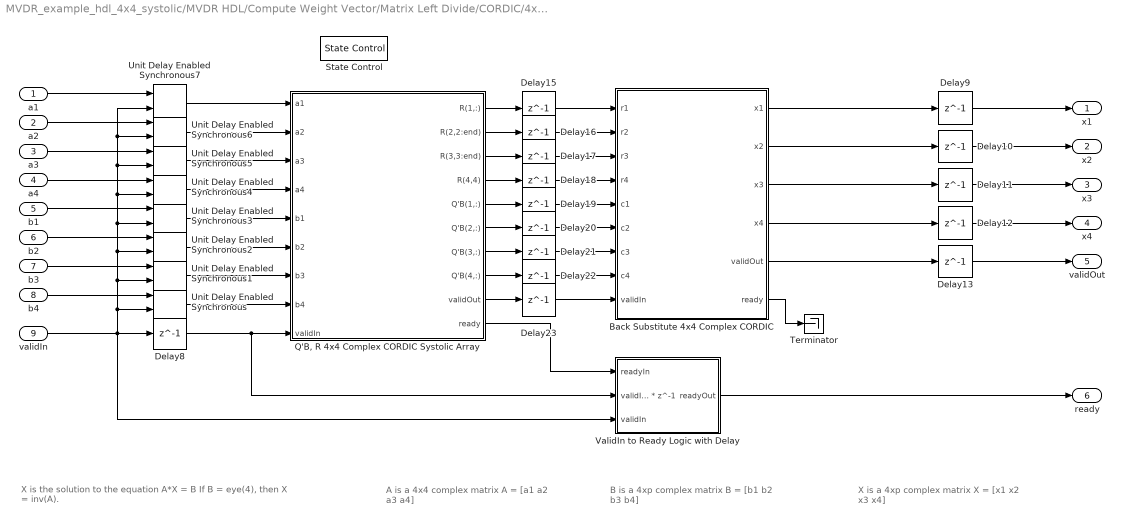
== system MVDR_example_hdl_4x4_systolic/MVDR HDL/Compute Weight Vector/Matrix Left Divide/CORDIC/4x4 Complex CORDIC Matrix Left Divide ==
  note: X is a 4xp complex matrix
      |
      | X = [x1
      | x2
      | x3
      | x4]
  note: B is a 4xp complex matrix
      |
      | B = [b1
      | b2
      | b3
      | b4]
  note: A is a 4x4 complex matrix
      |
      | A = [a1
      | a2
      | a3
      | a4]
  note: X is the solution to the equation A*X = B
      |
      | If B = eye(4), then X = inv(A).
  a1 : Inport
  a2 : Inport  Port=2
  a3 : Inport  Port=3
  a4 : Inport  Port=4
  b1 : Inport  Port=5
  b2 : Inport  Port=6
  b3 : Inport  Port=7
  b4 : Inport  Port=8
  validIn : Inport  Port=9
  Back Substitute 4x4 Complex CORDIC : Subsystem  TreatAsAtomicUnit=on  mask{NumberOfCORDICIterations=NumberOfCORDICIterations, OutputPrototype=OutputPrototype}
      mask prompts: NumberOfCORDICIterations "Number of CORDIC Iterations"; OutputPrototype "Output Prototype"
  Delay{8..13,15..23} (15 alike) : Delay  DelayLength=1
  "Q'B, R 4x4 Complex CORDIC Systolic Array" : Subsystem  TreatAsAtomicUnit=on  mask{NumberOfCORDICIterations=NumberOfCORDICIterations}
      mask prompts: NumberOfCORDICIterations "Number of CORDIC Iterations"
  State Control : StateControl  StateControl=Synchronous
  Terminator : Terminator
  Unit Delay Enabled Synchronous{,1..7} (8 alike) : hdlsllib/Discrete/Unit Delay Enabled Synchronous  InitialCondition=0.0  SampleTime=-1
      settings: SourceProductBaseCode=SL
  ValidIn to Ready Logic with Delay : Subsystem
  x1 : Outport  VectorParamsAs1DForOutWhenUnconnected=off
  x2 : Outport  Port=2  VectorParamsAs1DForOutWhenUnconnected=off
  x3 : Outport  Port=3  VectorParamsAs1DForOutWhenUnconnected=off
  x4 : Outport  Port=4  VectorParamsAs1DForOutWhenUnconnected=off
  validOut : Outport  Port=5  VectorParamsAs1DForOutWhenUnconnected=off
  ready : Outport  Port=6  VectorParamsAs1DForOutWhenUnconnected=off
  wires:
  "Q'B, R 4x4 Complex CORDIC Systolic Array"/10(ready) -> ValidIn to Ready Logic with Delay/1(readyIn)
  Delay23/1 -> Back Substitute 4x4 Complex CORDIC/9(validIn)
  Delay22/1 -> Back Substitute 4x4 Complex CORDIC/8(c4)
  Delay21/1 -> Back Substitute 4x4 Complex CORDIC/7(c3)
  Delay20/1 -> Back Substitute 4x4 Complex CORDIC/6(c2)
  Delay19/1 -> Back Substitute 4x4 Complex CORDIC/5(c1)
  Delay18/1 -> Back Substitute 4x4 Complex CORDIC/4(r4)
  Delay17/1 -> Back Substitute 4x4 Complex CORDIC/3(r3)
  Delay16/1 -> Back Substitute 4x4 Complex CORDIC/2(r2)
  Delay15/1 -> Back Substitute 4x4 Complex CORDIC/1(r1)
  Back Substitute 4x4 Complex CORDIC/6(ready) -> Terminator/1
  Back Substitute 4x4 Complex CORDIC/5(validOut) -> Delay13/1
  ValidIn to Ready Logic with Delay/1(readyOut) -> ready/1
  "Q'B, R 4x4 Complex CORDIC Systolic Array"/9(validOut) -> Delay23/1
  "Q'B, R 4x4 Complex CORDIC Systolic Array"/8(Q'B(4,:)) -> Delay22/1
  "Q'B, R 4x4 Complex CORDIC Systolic Array"/7(Q'B(3,:)) -> Delay21/1
  "Q'B, R 4x4 Complex CORDIC Systolic Array"/6(Q'B(2,:)) -> Delay20/1
  "Q'B, R 4x4 Complex CORDIC Systolic Array"/5(Q'B(1,:)) -> Delay19/1
  "Q'B, R 4x4 Complex CORDIC Systolic Array"/4(R(4,4)) -> Delay18/1
  "Q'B, R 4x4 Complex CORDIC Systolic Array"/3(R(3,3:end)) -> Delay17/1
  "Q'B, R 4x4 Complex CORDIC Systolic Array"/2(R(2,2:end)) -> Delay16/1
  "Q'B, R 4x4 Complex CORDIC Systolic Array"/1(R(1,:)) -> Delay15/1
  Back Substitute 4x4 Complex CORDIC/4(x4) -> Delay12/1
  Back Substitute 4x4 Complex CORDIC/3(x3) -> Delay11/1
  Back Substitute 4x4 Complex CORDIC/1(x1) -> Delay9/1
  Back Substitute 4x4 Complex CORDIC/2(x2) -> Delay10/1
  Delay13/1 -> validOut/1
  Delay12/1 -> x4/1
  Delay11/1 -> x3/1
  Delay10/1 -> x2/1
  Delay9/1 -> x1/1
  Unit Delay Enabled Synchronous7/1 -> "Q'B, R 4x4 Complex CORDIC Systolic Array"/1(a1)
  Unit Delay Enabled Synchronous6/1 -> "Q'B, R 4x4 Complex CORDIC Systolic Array"/2(a2)
  Unit Delay Enabled Synchronous5/1 -> "Q'B, R 4x4 Complex CORDIC Systolic Array"/3(a3)
  Unit Delay Enabled Synchronous4/1 -> "Q'B, R 4x4 Complex CORDIC Systolic Array"/4(a4)
  Unit Delay Enabled Synchronous3/1 -> "Q'B, R 4x4 Complex CORDIC Systolic Array"/5(b1)
  Unit Delay Enabled Synchronous2/1 -> "Q'B, R 4x4 Complex CORDIC Systolic Array"/6(b2)
  Unit Delay Enabled Synchronous1/1 -> "Q'B, R 4x4 Complex CORDIC Systolic Array"/7(b3)
  Unit Delay Enabled Synchronous/1 -> "Q'B, R 4x4 Complex CORDIC Systolic Array"/8(b4)
  Delay8/1 -> "Q'B, R 4x4 Complex CORDIC Systolic Array"/9(validIn), ValidIn to Ready Logic with Delay/2(validIn * z^-1)
  validIn/1 -> Delay8/1, ValidIn to Ready Logic with Delay/3(validIn), Unit Delay Enabled Synchronous7/2, Unit Delay Enabled Synchronous6/2, Unit Delay Enabled Synchronous5/2, Unit Delay Enabled Synchronous4/2, Unit Delay Enabled Synchronous3/2, Unit Delay Enabled Synchronous2/2, Unit Delay Enabled Synchronous1/2, Unit Delay Enabled Synchronous/2
  b4/1 -> Unit Delay Enabled Synchronous/1
  b3/1 -> Unit Delay Enabled Synchronous1/1
  b2/1 -> Unit Delay Enabled Synchronous2/1
  b1/1 -> Unit Delay Enabled Synchronous3/1
  a4/1 -> Unit Delay Enabled Synchronous4/1
  a3/1 -> Unit Delay Enabled Synchronous5/1
  a2/1 -> Unit Delay Enabled Synchronous6/1
  a1/1 -> Unit Delay Enabled Synchronous7/1

== system MVDR_example_hdl_4x4_systolic/MVDR HDL/Compute Weight Vector/Matrix Left Divide/QR Solver/Emulate CORDIC Ready ==
  In1 : Inport
  Compare To Constant : simulink/Logic and Bit Operations/Compare To Constant  relop===  const=NumberOfCORDICIterations+7  OutDataTypeStr=boolean
  Compare To Zero : simulink/Logic and Bit Operations/Compare To Zero  relop===  OutDataTypeStr=boolean
  Compare To Zero1 : simulink/Logic and Bit Operations/Compare To Zero  relop=>  OutDataTypeStr=boolean
  HDL Counter : hdlsllib/Sources/HDL Counter  CountType=Free running  CountInit=0  CountStep=1  CountMax=25  CountFromType=Initial value  CountFrom=0  CountResetPort=on  CountLoadPort=off  CountEnbPort=on  CountDirPort=off  CountDataType=Unsigned  CountWordLen=32  CountFracLen=0  CountSampTime=1
  Logical Operator : Logic  Operator=OR  AllPortsSameDT=off  OutDataTypeStr=boolean
  Out1 : Outport
  wires:
  HDL Counter/1 -> Compare To Zero1/1, Compare To Constant/1, Compare To Zero/1
  Compare To Constant/1 -> HDL Counter/1
  Compare To Zero1/1 -> Logical Operator/2
  Logical Operator/1 -> HDL Counter/2
  In1/1 -> Logical Operator/1
  Compare To Zero/1 -> Out1/1

== system MVDR_example_hdl_4x4_systolic/MVDR HDL/Compute Weight Vector/Matrix Left Divide/QR Solver/Subsystem ==
  In1 : Inport
  In2 : Inport  Port=2
  Enable : EnablePort
  QR Solver : dspsolvers/QR Solver  SimulateUsing=Interpreted execution
      settings: SourceProductBaseCode=DS
  Out1 : Outport
  wires:
  In2/1 -> QR Solver/2
  QR Solver/1 -> Out1/1
  In1/1 -> QR Solver/1

== system MVDR_example_hdl_4x4_systolic/MVDR HDL/Form Covariance Matrix/Matrix Multiply Partitioned/Partition x_conj/Partition x ==
  x : Inport  Partition=on  PartitionDimension=1  PartitionWidth=1  PartitionOffset=0
  x_conj_elem : Inport  Port=2
  For Each : ForEach  DisableCoverage=on
  HDL Complex Multiply : Subsystem  mask(HDL Complex Multiplier (3 Multiply, 5 Add)){D1=2, D2=1, D3=1, D4=1, D5=1}
      mask help:
      | Xilinx devices:
      | - Set D1 = 1 or 2 to trade off speed & FF resources
      | - Set D2-D5 = 1 to fully leverage DSP48 pipelines
      | - Use sync reset
      |
      | Intel FPGAs:
      | - Set D1 = 1 or 2 depending on device family
      | - Set D5 = 1; D2, D3, D4 = 0
      | - Use async reset
      mask init:
      | delay = D1+D2+D3+D4+D5;
      mask Display:
      | fprintf('Delay=%d',delay);
      | port_label('input',1,'z1');
      | port_label('input',2,'z2');
  C_col : Outport  ConcatenationDimension=1
  wires:
  x/1 -> HDL Complex Multiply/1(In1)
  x_conj_elem/1 -> HDL Complex Multiply/2(In2)
  HDL Complex Multiply/1(Out1) -> C_col/1

== system MVDR_example_hdl_4x4_systolic/MVDR HDL/Normalize Response/MVDR Weight Update/Inner Product/Element-wise complex product ==
  u : Inport  Partition=on  PartitionDimension=1  PartitionWidth=1  PartitionOffset=0
  v : Inport  Port=2  Partition=on  PartitionDimension=1  PartitionWidth=1  PartitionOffset=0
  For Each : ForEach  DisableCoverage=on
  HDL Complex Multiply : Subsystem  mask(HDL Complex Multiplier (3 Multiply, 5 Add)){D1=2, D2=1, D3=1, D4=1, D5=1}
      mask help:
      | Xilinx devices:
      | - Set D1 = 1 or 2 to trade off speed & FF resources
      | - Set D2-D5 = 1 to fully leverage DSP48 pipelines
      | - Use sync reset
      |
      | Intel FPGAs:
      | - Set D1 = 1 or 2 depending on device family
      | - Set D5 = 1; D2, D3, D4 = 0
      | - Use async reset
      mask init:
      | delay = D1+D2+D3+D4+D5;
      mask Display:
      | fprintf('Delay=%d',delay);
      | port_label('input',1,'z1');
      | port_label('input',2,'z2');
  y : Outport  ConcatenationDimension=1
  wires:
  v/1 -> HDL Complex Multiply/2(In2)
  HDL Complex Multiply/1(Out1) -> y/1
  u/1 -> HDL Complex Multiply/1(In1)

== system MVDR_example_hdl_4x4_systolic/MVDR HDL/Normalize Response/MVDR Weight Update/Inner Product/Tree Sum with Distributed Pipelining ==
  In1 : Inport
  Delay3 : Delay  DelayLength=ceil(log2(numArrayElements))
  Tree Sum of Elements : Sum  Inputs=+  OutDataTypeStr=Inherit: Same as first input  LockScale=on
  Out1 : Outport
  wires:
  Delay3/1 -> Out1/1
  In1/1 -> Tree Sum of Elements/1
  Tree Sum of Elements/1 -> Delay3/1
